simulink library "adptfiltsubsys"  (Simulink 8.0)
settings: Solver=ode45  SolverMode=SingleTasking  StartTime=0.0  StopTime=10.0  RelTol=1e-3
values from neighbouring files (symbols this model uses):
  L = h.Length    [maxstep.m]    (also in msepred.m; msesim.m)
  N = str2double(s)    [dspcsum.m]    (also in dspddes3Transform.m = sprintf('; dspwdes.m = varargin{2}; if isempty(N), N=64; end)
undefined symbols (not defined in the file or in its folder): leakage, Radix
libraries: dspxfrm3 x5, dspsigops x3, dspmtrx3 x2, adptfiltsubsys x1
settings Model: FPTRunName=Active  Creator=navan  LastModifiedBy=lij

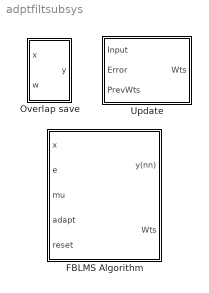
== system adptfiltsubsys ==
  FBLMS Algorithm : Subsystem  mask(FBLMS Algorithm){weights_algo=on}
      mask prompts: weights_algo "Output filter weights"
      mask help: Fast Block LMS algorithm using FFT.
      mask init:
      | dspblkblmsalgo('fblms');
  Overlap save : Subsystem
  Update : Subsystem  mask(LMS based weight updates){Algo=LMS, stepflag=Dialog box, mu=0.1, leakage=1.0, Adapt=off, icw=0}
      mask prompts: Algo "Algorithm:"; stepflag "Specify step-size via:"; mu "Step-size, mu:"; leakage "Leakage factor (0 to 1):"; Adapt "Enable/disable adaptation via input port"; icw "Initial value of filter weights:"
      mask help: Weight update equlation for LMS based filters.
      mask init:
      | s=dspblklmsupdate('init');
      mask StyleString: popup(LMS|Normalized LMS|Sign-Error LMS|Sign-Data LMS|Sign-Sign LMS),popup(Dialog box|Input port),edit,edit,checkbox,edit
      mask CallbackString: |dspblklmsupdate('stepflag');|||dspblklmsupdate('init');|
      mask Display: disp(s);

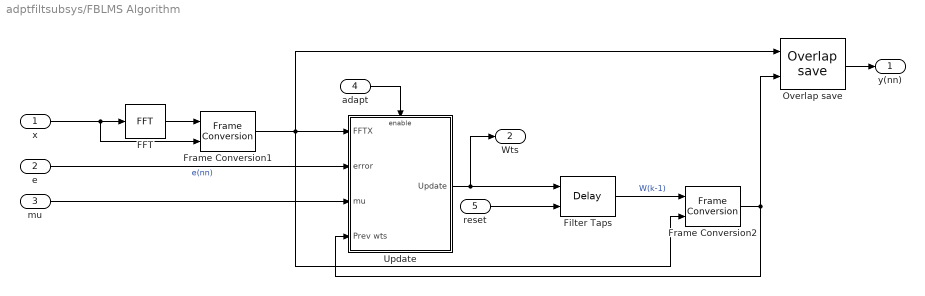
== system adptfiltsubsys/FBLMS Algorithm ==
  x : Inport
  e : Inport  Port=2
  mu : Inport  Port=3
  adapt : Inport  Port=4
  reset : Inport  Port=5
  FFT : dspxfrm3/FFT  CompMethod=Table lookup  TableOpt=NEW  TableOptActive=Speed  BitRevOrder=off  InheritFFTLength=on  FFTLength=64  RowConvenienceOn=on  FFTImplementation=Radix-2  SkipNorm=off  firstCoeffDataTypeStr=Inherit: Same word length as input  firstCoeffLastDataTypeStr=Inherit: Same word length as input  outputMin=[]  outputMax=[]  roundingMode=Floor  overflowMode=off
  Filter Taps : dspsigops/Delay  InputProcessing=Columns as channels (frame based)  dly_unit=Samples  delay=L  ic_detail=on  dif_ic_for_ch=off  dif_ic_for_dly=off  ic=ic  reset_popup=Non-zero sample
  Frame Conversion1 : FrameConversion  InheritSamplingMode=on
  Frame Conversion2 : FrameConversion  InheritSamplingMode=on
  Overlap save : adptfiltsubsys/Overlap save
  Update : Subsystem
  y(nn) : Outport
  Wts : Outport  Port=2
  wires:
  FFT/1 -> Frame Conversion1/1
  Frame Conversion1/1 -> Overlap save/1, Update/1(FFTX), Frame Conversion2/2
  reset/1 -> Filter Taps/2
  adapt/1 -> Update/Enable
  e/1 -> Update/2(error)  "e(nn)"
  Update/1(Update) -> Wts/1, Filter Taps/1
  x/1 -> FFT/1, Frame Conversion1/2
  mu/1 -> Update/3(mu)
  Overlap save/1 -> y(nn)/1
  Filter Taps/1 -> Frame Conversion2/1  "W(k-1)"
  Frame Conversion2/1 -> Overlap save/2, Update/4(Prev wts)

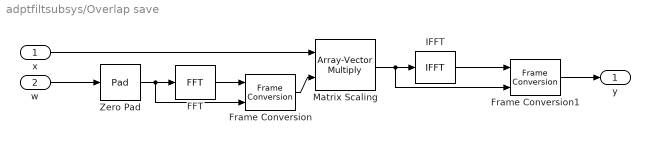
== system adptfiltsubsys/Overlap save ==
  x : Inport
  w : Inport  Port=2
  FFT : dspxfrm3/FFT  CompMethod=Table lookup  TableOpt=NEW  TableOptActive=Speed  BitRevOrder=off  InheritFFTLength=on  FFTLength=64  SkipNorm=off  firstCoeffDataTypeStr=Inherit: Same word length as input  firstCoeffLastDataTypeStr=Inherit: Same word length as input  outputMin=[]  outputMax=[]  roundingMode=Floor  overflowMode=off
  Frame Conversion : FrameConversion  InheritSamplingMode=on
  Frame Conversion1 : FrameConversion  InheritSamplingMode=on
  IFFT : dspxfrm3/IFFT  CompMethod=Table lookup  TableOpt=HYBRID  TableOptActive=Speed  BitRevOrder=off  cs_in=off  SkipNorm=on  InheritFFTLength=on  FFTLength=64  mode=Real  outSamplingMode=Frame based  firstCoeffDataTypeStr=Inherit: Same word length as input  firstCoeffLastDataTypeStr=Inherit: Same word length as input  outputMin=[]  outputMax=[]  roundingMode=Floor  overflowMode=off
  Matrix Scaling : dspmtrx3/Array-Vector Multiply  mode=Mute  saveAsFlag=0  Dimension=1  V_Source=Input port  V_VectFromMask=[0.5 0.25]  firstCoeffDataTypeStr=Inherit: Same word length as input  firstCoeffLastDataTypeStr=Inherit: Same word length as input  firstCoeffMin=[]  firstCoeffMax=[]  outputDataTypeStr=Inherit: Same as product output  outputLastDataTypeStr=Inherit: Same as product output  outputMin=[]  outputMax=[]  roundingMode=Floor  overflowMode=off
  Zero Pad : dspsigops/Pad  padAlong=Columns  dimsToPad=1  valSrc=Specify via dialog  padVal=0  spec=Output size  padNumOutRowsSpecMethod=User-specified  numOutRows=L+N  padNumOutColsSpecMethod=User-specified  numOutCols=1  isVarDimsMode=off  padBeginning=0  padEnd=0  outSizeMode=User-specified  outSize=1  padSigAt=End  trunc_flag=None  roundingMode=Floor  overflowMode=off  truncOrWrapMode=Truncate  wrap_flag=None
  y : Outport
  wires:
  IFFT/1 -> Frame Conversion1/1
  Frame Conversion1/1 -> y/1
  FFT/1 -> Frame Conversion/1
  Frame Conversion/1 -> Matrix Scaling/2
  w/1 -> Zero Pad/1
  Zero Pad/1 -> FFT/1, Frame Conversion/2
  x/1 -> Matrix Scaling/1
  Matrix Scaling/1 -> IFFT/1, Frame Conversion1/2

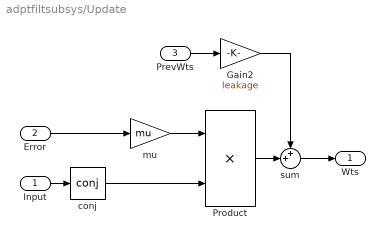
== system adptfiltsubsys/Update ==
  Input : Inport
  Error : Inport  Port=2
  PrevWts : Inport  Port=3
  Gain2 : Gain  Gain=leakage  SaturateOnIntegerOverflow=on  OutDataTypeStr=Inherit: Same as input  ParamDataTypeStr=Inherit: Same as input
  Product : Product  SaturateOnIntegerOverflow=on
  conj : Math  Operator=conj  SaturateOnIntegerOverflow=on
  mu : Gain  Gain=mu  SaturateOnIntegerOverflow=on  OutDataTypeStr=Inherit: Same as input  ParamDataTypeStr=Inherit: Same as input
  sum : Sum  Inputs=++|  SaturateOnIntegerOverflow=on  InputSameDT=on  OutDataTypeStr=Inherit: Same as first input
  Wts : Outport  InitialOutput=icw(:)
  wires:
  mu/1 -> Product/1
  Error/1 -> mu/1
  conj/1 -> Product/2
  Input/1 -> conj/1
  sum/1 -> Wts/1
  Product/1 -> sum/2
  PrevWts/1 -> Gain2/1
  Gain2/1 -> sum/1

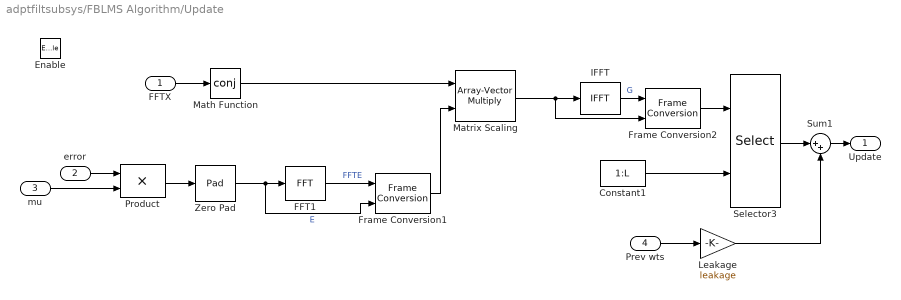
== system adptfiltsubsys/FBLMS Algorithm/Update ==
  FFTX : Inport
  error : Inport  Port=2
  mu : Inport  Port=3
  Prev wts : Inport  Port=4
  Enable : EnablePort
  Constant1 : Constant  Value=1:L
  FFT1 : dspxfrm3/FFT  CompMethod=Table lookup  TableOpt=NEW  TableOptActive=Speed  BitRevOrder=off  InheritFFTLength=on  FFTLength=64  RowConvenienceOn=on  FFTImplementation=Auto  SkipNorm=off  firstCoeffDataTypeStr=Inherit: Same word length as input  firstCoeffLastDataTypeStr=Inherit: Same word length as input  outputMin=[]  outputMax=[]  accumDataTypeStr=Inherit: Same as product output  accumLastDataTypeStr=Inherit: Same as product output  roundingMode=Floor  overflowMode=off
  Frame Conversion1 : FrameConversion  InheritSamplingMode=on
  Frame Conversion2 : FrameConversion  InheritSamplingMode=on
  IFFT : dspxfrm3/IFFT  CompMethod=Table lookup  TableOpt=HYBRID  TableOptActive=Speed  BitRevOrder=off  cs_in=off  SkipNorm=on  InheritFFTLength=on  FFTLength=64  mode=Real  outSamplingMode=Frame based  RowConvenienceOn=on  FFTImplementation=Auto  firstCoeffDataTypeStr=Inherit: Same word length as input  firstCoeffLastDataTypeStr=Inherit: Same word length as input  outputMin=[]  outputMax=[]  accumDataTypeStr=Inherit: Same as product output  accumLastDataTypeStr=Inherit: Same as product output  roundingMode=Floor  overflowMode=off
  Leakage : Gain  Gain=leakage  SaturateOnIntegerOverflow=on  OutDataTypeStr=Inherit: Same as input  ParamDataTypeStr=Inherit: Same as input
  Math Function : Math  Operator=conj  SaturateOnIntegerOverflow=on
  Matrix Scaling : dspmtrx3/Array-Vector Multiply  mode=Mute  saveAsFlag=0  Dimension=1  V_Source=Input port  V_VectFromMask=[0.5 0.25]  firstCoeffSignedness=Auto  firstCoeffDataTypeStr=Inherit: Same word length as input  firstCoeffLastDataTypeStr=Inherit: Same word length as input  firstCoeffMin=[]  firstCoeffMax=[]  outputSignedness=Auto  outputDataTypeStr=Inherit: Same as product output  outputLastDataTypeStr=Inherit: Same as product output  outputMin=[]  outputMax=[]  accumSignedness=Auto  prodOutputSignedness=Auto  roundingMode=Floor  overflowMode=off
  Product : Product  SaturateOnIntegerOverflow=on  InputSameDT=on  OutDataTypeStr=Inherit: Same as first input
  Selector3 : Selector  IndexOptions=Index vector (port)  Indices=[1 3]  OutputSizes=1
  Sum1 : Sum  Inputs=|++  SaturateOnIntegerOverflow=on
  Zero Pad : dspsigops/Pad  padAlong=Columns  dimsToPad=1  valSrc=Specify via dialog  padVal=0  spec=Output size  padNumOutRowsSpecMethod=User-specified  numOutRows=L+N  padNumOutColsSpecMethod=User-specified  numOutCols=1  isVarDimsMode=off  padBeginning=0  padEnd=0  outSizeMode=User-specified  outSize=1  padSigAt=Beginning  trunc_flag=Error  roundingMode=Floor  overflowMode=off  truncOrWrapMode=Truncate  wrap_flag=None
  Update : Outport
  wires:
  FFT1/1 -> Frame Conversion1/1  "FFTE"
  Frame Conversion1/1 -> Matrix Scaling/2
  FFTX/1 -> Math Function/1
  Constant1/1 -> Selector3/2
  Matrix Scaling/1 -> IFFT/1, Frame Conversion2/2
  Math Function/1 -> Matrix Scaling/1
  Zero Pad/1 -> FFT1/1, Frame Conversion1/2  "E"
  Prev wts/1 -> Leakage/1
  Leakage/1 -> Sum1/2
  Selector3/1 -> Sum1/1
  Sum1/1 -> Update/1
  error/1 -> Product/1
  mu/1 -> Product/2
  Product/1 -> Zero Pad/1
  Frame Conversion2/1 -> Selector3/1
  IFFT/1 -> Frame Conversion2/1  "G"
